simulink model "AdaptiveControlEg"  (R2020b)
settings: Solver=VariableStepAuto  StartTime=0.0  StopTime=10.0  RelTol=1e-3
values from neighbouring files (symbols this model uses):
  Gamma = diag([1,1])    [param.m]
  gamma = 10    [param.m]
  P = lyap(A_m, Q)    [param.m]
  para_m = [ratio_m, w_m]    [param.m]
libraries: simulink x1
settings Model: Creator=vicgd  LastModifiedBy=vicgd

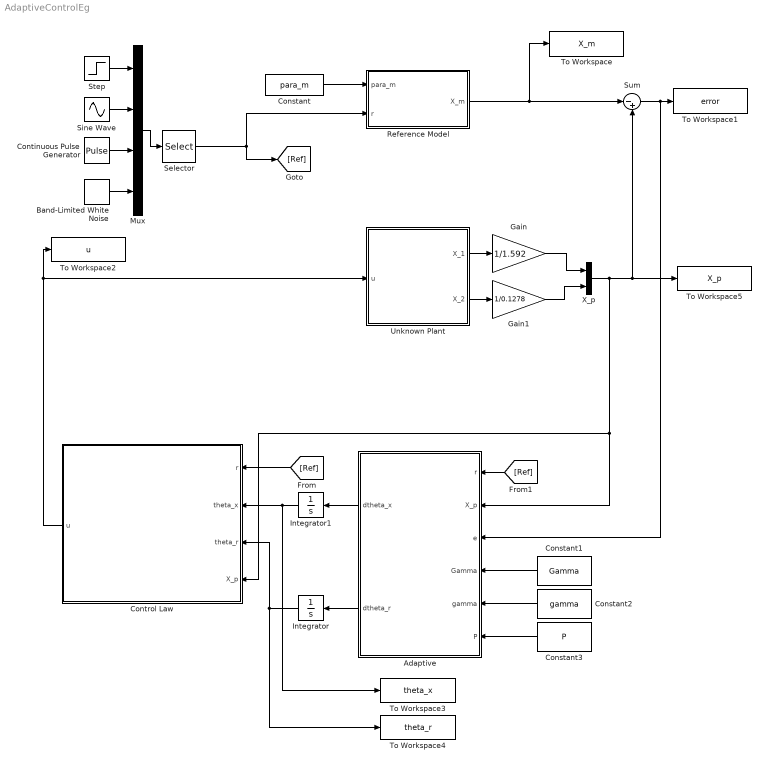
== system AdaptiveControlEg ==
  Adaptive : MATLAB Function  TreatAsAtomicUnit=on
  Band-Limited White Noise : simulink/Sources/Band-Limited White Noise  Cov=[1]  Ts=0.1  seed=[23341]
  Constant : Constant  Value=para_m
  Constant1 : Constant  Value=Gamma
  Constant2 : Constant  Value=gamma
  Constant3 : Constant  Value=P
  Continuous Pulse Generator : DiscretePulseGenerator  PulseType=Time based  Period=0.5  PulseWidth=50
  Control Law : MATLAB Function  TreatAsAtomicUnit=on
  Gain : Gain  Gain=1/1.592
  Gain1 : Gain  Gain=1/0.1278
  Integrator : Integrator
  Integrator1 : Integrator
  Mux : Mux
  Reference Model : Subsystem
  Selector : Selector  InputPortWidth=4  IndexOptions=Index vector (dialog)  Indices=[2]  OutputSizes=1
  Sine Wave : Sin  Frequency=10  SampleTime=0
  Step : Step  SampleTime=0
  Sum : Sum  Inputs=|-+
  To Workspace : ToWorkspace  VariableName=X_m  SaveFormat=Timeseries  SampleTime=-1
  To Workspace1 : ToWorkspace  VariableName=error  SaveFormat=Timeseries  SampleTime=-1
  To Workspace2 : ToWorkspace  VariableName=u  SaveFormat=Timeseries  SampleTime=-1
  To Workspace3 : ToWorkspace  VariableName=theta_x  SaveFormat=Timeseries  SampleTime=-1
  To Workspace4 : ToWorkspace  VariableName=theta_r  SaveFormat=Timeseries  SampleTime=-1
  To Workspace5 : ToWorkspace  VariableName=X_p  SaveFormat=Timeseries  SampleTime=-1
  Unknown Plant : Subsystem
  X_p : Mux  Inputs=2
  wires:
  Unknown Plant/1(X_1) -> Gain/1
  Unknown Plant/2(X_2) -> Gain1/1
  Reference Model/1(X_m) -> To Workspace/1, Sum/1
  X_p/1 -> Control Law/4(X_p), Adaptive/2(X_p), To Workspace5/1, Sum/2
  Sum/1 -> To Workspace1/1, Adaptive/3(e)
  Constant1/1 -> Adaptive/4(Gamma)
  Constant2/1 -> Adaptive/5(gamma)
  Constant3/1 -> Adaptive/6(P)
  Integrator1/1 -> Control Law/2(theta_x), To Workspace3/1
  Integrator/1 -> Control Law/3(theta_r), To Workspace4/1
  Adaptive/2(dtheta_r) -> Integrator/1
  Adaptive/1(dtheta_x) -> Integrator1/1
  Gain/1 -> X_p/1
  Gain1/1 -> X_p/2
  Constant/1 -> Reference Model/1(para_m)
  Control Law/1(u) -> To Workspace2/1, Unknown Plant/1(u)
  [Ref] -> Control Law/1(r)
  [Ref] -> Adaptive/1(r)
  Continuous Pulse Generator/1 -> Mux/3
  Selector/1 -> Reference Model/2(r), [Ref]
  Step/1 -> Mux/1
  Sine Wave/1 -> Mux/2
  Mux/1 -> Selector/1
  Band-Limited White Noise/1 -> Mux/4

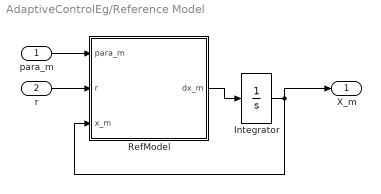
== system AdaptiveControlEg/Reference Model ==
  para_m : Inport
  r : Inport  Port=2
  Integrator : Integrator  InitialCondition=[0 0]
  RefModel : MATLAB Function  TreatAsAtomicUnit=on
  X_m : Outport
  wires:
  Integrator/1 -> X_m/1, RefModel/3(x_m)
  RefModel/1(dx_m) -> Integrator/1
  r/1 -> RefModel/2(r)
  para_m/1 -> RefModel/1(para_m)

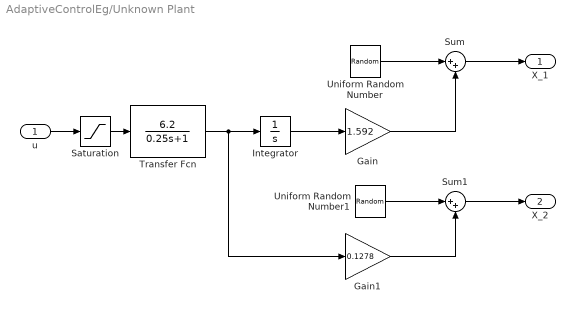
== system AdaptiveControlEg/Unknown Plant ==
  u : Inport
  Gain : Gain  Gain=1.592
  Gain1 : Gain  Gain=0.1278
  Integrator : Integrator
  Saturation : Saturate  UpperLimit=5  LowerLimit=-5  LinearizeAsGain=off
  Sum : Sum  Inputs=|++
  Sum1 : Sum  Inputs=|++
  Transfer Fcn : TransferFcn  Numerator=[6.2]  Denominator=[0.25 1]
  Uniform Random Number : UniformRandomNumber  Minimum=-0.001  Maximum=0.001  SampleTime=0.1
  Uniform Random Number1 : UniformRandomNumber  Minimum=-0.001  Maximum=0.001  SampleTime=0.1
  X_1 : Outport
  X_2 : Outport  Port=2
  wires:
  u/1 -> Saturation/1
  Uniform Random Number/1 -> Sum/1
  Saturation/1 -> Transfer Fcn/1
  Integrator/1 -> Gain/1
  Gain1/1 -> Sum1/2
  Gain/1 -> Sum/2
  Sum/1 -> X_1/1
  Sum1/1 -> X_2/1
  Transfer Fcn/1 -> Integrator/1, Gain1/1
  Uniform Random Number1/1 -> Sum1/1

== matlab function AdaptiveControlEg/Adaptive ==
  data: r input; dtheta_x output; X_p input; e input; Gamma input; gamma input; P input; dtheta_r output
function [dtheta_x, dtheta_r] = Adaptive(r,X_p,e,Gamma,gamma,P)
sgn_g   = 1; 
b       = [0;1];

dtheta_x = -sgn_g * Gamma * (e.'*P*b)*X_p;
dtheta_r = -sgn_g * gamma * (e.'*P*b)*r;

== matlab function AdaptiveControlEg/Reference Model/RefModel ==
  data: para_m input; dx_m output; r input; x_m input
function dx_m = RefModel(para_m,r,x_m)
ratio_m = para_m(1);
w_m     = para_m(2);
A_m     = [0, 1;
           -w_m^2, -2*ratio_m*w_m];
b       = [0; 1];
g_m     = w_m^2;
dx_m    = (A_m*x_m)+(g_m*b*r);

== matlab function AdaptiveControlEg/Control Law ==
  data: r input; u output; theta_x input; theta_r input; X_p input
function u = Ctrl(r, theta_x, theta_r, X_p)
u = theta_x.' * X_p + theta_r * r;
